simulink model "fblin_singletrack_lopez2"  (R2018b)
settings: Solver=VariableStepAuto  StartTime=0.0  StopTime=5.0  RelTol=1e-3
values from neighbouring files (symbols this model uses):
  actuation_delay = 0.09    [init_singletrack.m]
  beta_velocity_threshold = 0.05    [init_singletrack.m]
  car_param = [a, b, Cf, Cr, Iz, m]    [init_singletrack.m]
  car_state0 = [psi0, r0, beta0, x0, y0]    [init_singletrack.m]
  fblin_Ts = 0.01    [init_singletrack.m]
  meas_Ts = 0.001    [init_singletrack.m]
  P = 0.5    [init_singletrack.m]    (also in init_unicycle.m)
  psi_fir = [0.0144, 0.0439, 0.1202, 0.2025, 0.2380, 0.2025, 0.1202, 0.0439, 0.0144]    [init_singletrack.m]
  psi_noiseVar = 9e-7    (= 9e-07)    [init_singletrack.m]
  r_noiseVar = 9e-7    (= 9e-07)    [init_singletrack.m]
  vel_fir = [0.0144, 0.0295, 0.0763, 0.0823, 0.0355, -0.0355, -0.0823, -0.0763, -0.0295, -0.0144]    [init_singletrack.m]
  xy_noiseVar = 1e-8    (= 1e-08)    [init_singletrack.m]
undefined symbols (not defined in the file or in its folder): DiscIntNeverNeededParam, fblin_control_singletrack_lopez2, fblin_output_singletrack_lopez2, sigmf, singleTrack_model
libraries: simulink x1
settings Model: Creator=bascetta  LastModifiedBy=bascetta
settings DebuggingCC: LibraryContextMissingDiagnostic=none
settings SFSimCC: SimUseLocalCustomCode=off
settings RTWCC: RTWUseLocalCustomCode=off

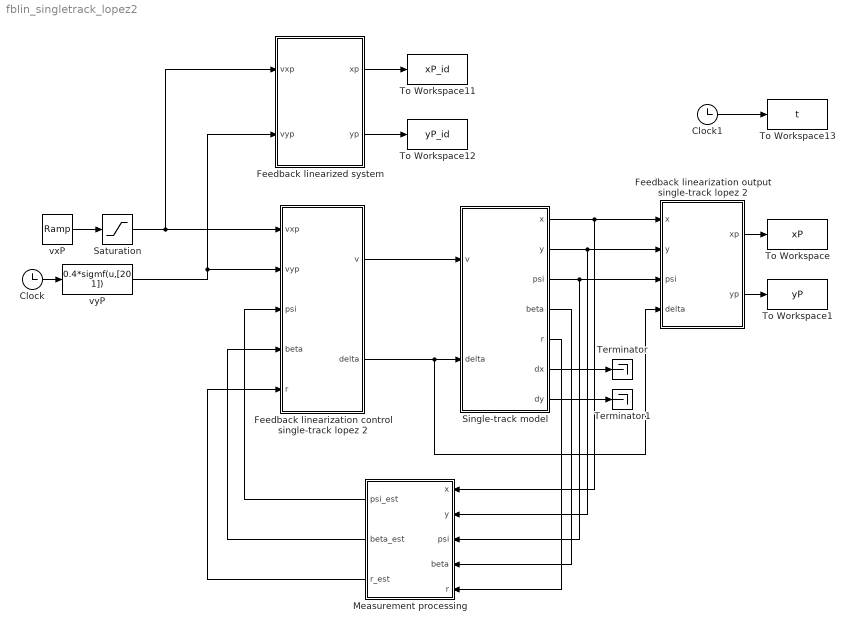
== system fblin_singletrack_lopez2 ==
  Clock : Clock
  Clock1 : Clock
  Feedback linearization control single-track lopez 2 : Subsystem  mask{car_parameters=car_param, P_dist=P, Ts=fblin_Ts}
      mask prompts: car_parameters "Car parameters"; P_dist "Distance of point P"; Ts "Sampling time"
  Feedback linearization output single-track lopez 2 : Subsystem  mask{car_parameters=car_param, P_dist=P}
      mask prompts: car_parameters "Car parameters"; P_dist "Distance of point P"
  Feedback linearized system : Subsystem  mask{car_parameters=car_param, car_initial_state=car_state0, P_dist=P}
      mask prompts: car_parameters "Car parameters"; car_initial_state "Car initial state"; P_dist "Distance of point P"
  Measurement processing : Subsystem
  Saturation : Saturate  UpperLimit=0.4  LowerLimit=0.0
  Single-track model : Subsystem  mask{car_parameters=car_param, actuation_delay=actuation_delay}
      mask prompts: car_parameters "Car parameters"; actuation_delay "Actuation delay"
  Terminator : Terminator
  Terminator1 : Terminator
  To Workspace : ToWorkspace  VariableName=xP  SampleTime=meas_Ts
      settings: Save2DSignal=2-D array (concatenate along first dimension)
  To Workspace1 : ToWorkspace  VariableName=yP  SampleTime=meas_Ts
      settings: Save2DSignal=2-D array (concatenate along first dimension)
  To Workspace11 : ToWorkspace  VariableName=xP_id  SampleTime=meas_Ts
      settings: Save2DSignal=2-D array (concatenate along first dimension)
  To Workspace12 : ToWorkspace  VariableName=yP_id  SampleTime=meas_Ts
      settings: Save2DSignal=2-D array (concatenate along first dimension)
  To Workspace13 : ToWorkspace  VariableName=t  SampleTime=meas_Ts
      settings: Save2DSignal=2-D array (concatenate along first dimension)
  vxP : simulink/Sources/Ramp  slope=0.8  start=0  InitialOutput=0
  vyP : MATLABFcn  MATLABFcn=0.4*sigmf(u,[20 1])
  wires:
  Saturation/1 -> Feedback linearization control single-track lopez 2/1(vxp), Feedback linearized system/1(vxp)
  Feedback linearization output single-track lopez 2/2(yp) -> To Workspace1/1
  Feedback linearization output single-track lopez 2/1(xp) -> To Workspace/1
  Feedback linearized system/1(xp) -> To Workspace11/1
  Feedback linearized system/2(yp) -> To Workspace12/1
  Clock1/1 -> To Workspace13/1
  Single-track model/1(x) -> Measurement processing/1(x), Feedback linearization output single-track lopez 2/1(x)
  Single-track model/2(y) -> Measurement processing/2(y), Feedback linearization output single-track lopez 2/2(y)
  Single-track model/3(psi) -> Measurement processing/3(psi), Feedback linearization output single-track lopez 2/3(psi)
  Single-track model/4(beta) -> Measurement processing/4(beta)
  Feedback linearization control single-track lopez 2/2(delta) -> Feedback linearization output single-track lopez 2/4(delta), Single-track model/2(delta)
  Feedback linearization control single-track lopez 2/1(v) -> Single-track model/1(v)
  Single-track model/5(r) -> Measurement processing/5(r)
  Measurement processing/1(psi_est) -> Feedback linearization control single-track lopez 2/3(psi)
  Measurement processing/2(beta_est) -> Feedback linearization control single-track lopez 2/4(beta)
  Measurement processing/3(r_est) -> Feedback linearization control single-track lopez 2/5(r)
  Single-track model/7(dy) -> Terminator1/1
  Single-track model/6(dx) -> Terminator/1
  vxP/1 -> Saturation/1
  Clock/1 -> vyP/1
  vyP/1 -> Feedback linearized system/2(vyp), Feedback linearization control single-track lopez 2/2(vyp)

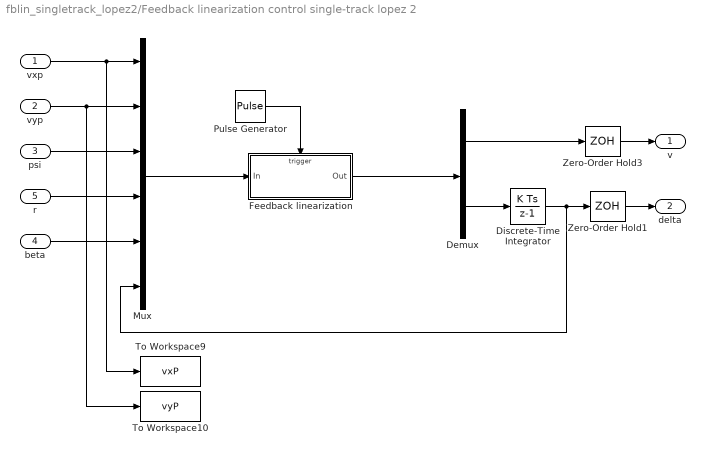
== system fblin_singletrack_lopez2/Feedback linearization control single-track lopez 2 ==
  vxp : Inport
  vyp : Inport  Port=2
  psi : Inport  Port=3
  beta : Inport  Port=4
  r : Inport  Port=5
  Demux : Demux  Outputs=2
  Discrete-Time Integrator : DiscreteIntegrator  SampleTime=Ts  ICPrevOutput=DiscIntNeverNeededParam  ICPrevScaledInput=DiscIntNeverNeededParam
  Feedback linearization : Subsystem  TreatAsAtomicUnit=on
  Mux : Mux  Inputs=6
  Pulse Generator : DiscretePulseGenerator  PulseType=Time based  Period=Ts  PulseWidth=50
  To Workspace10 : ToWorkspace  VariableName=vyP  SampleTime=meas_Ts
      settings: Save2DSignal=2-D array (concatenate along first dimension)
  To Workspace9 : ToWorkspace  VariableName=vxP  SampleTime=meas_Ts
      settings: Save2DSignal=2-D array (concatenate along first dimension)
  Zero-Order Hold1 : ZeroOrderHold  SampleTime=Ts
  Zero-Order Hold3 : ZeroOrderHold  SampleTime=Ts
  v : Outport
  delta : Outport  Port=2
  wires:
  vyp/1 -> To Workspace10/1, Mux/2
  Demux/1 -> Zero-Order Hold3/1
  vxp/1 -> To Workspace9/1, Mux/1
  psi/1 -> Mux/3
  beta/1 -> Mux/5
  r/1 -> Mux/4
  Zero-Order Hold3/1 -> v/1
  Discrete-Time Integrator/1 -> Mux/6, Zero-Order Hold1/1
  Zero-Order Hold1/1 -> delta/1
  Feedback linearization/1(Out) -> Demux/1
  Mux/1 -> Feedback linearization/1(In)
  Pulse Generator/1 -> Feedback linearization/Trigger
  Demux/2 -> Discrete-Time Integrator/1

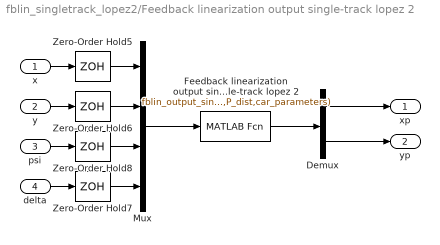
== system fblin_singletrack_lopez2/Feedback linearization output single-track lopez 2 ==
  x : Inport
  y : Inport  Port=2
  psi : Inport  Port=3
  delta : Inport  Port=4
  Demux : Demux  Outputs=2
  Feedback linearization output single-track lopez 2 : MATLABFcn  MATLABFcn=fblin_output_singletrack_lopez2(u(1),u(2),u(3),u(4),P_dist,car_parameters)  OutputDimensions=2
  Mux : Mux
  Zero-Order Hold{5..8} (4 alike) : ZeroOrderHold  SampleTime=fblin_Ts
  xp : Outport
  yp : Outport  Port=2
  wires:
  y/1 -> Zero-Order Hold6/1
  Demux/2 -> yp/1
  Feedback linearization output single-track lopez 2/1 -> Demux/1
  Demux/1 -> xp/1
  Mux/1 -> Feedback linearization output single-track lopez 2/1
  x/1 -> Zero-Order Hold5/1
  delta/1 -> Zero-Order Hold7/1
  psi/1 -> Zero-Order Hold8/1
  Zero-Order Hold5/1 -> Mux/1
  Zero-Order Hold6/1 -> Mux/2
  Zero-Order Hold7/1 -> Mux/4
  Zero-Order Hold8/1 -> Mux/3

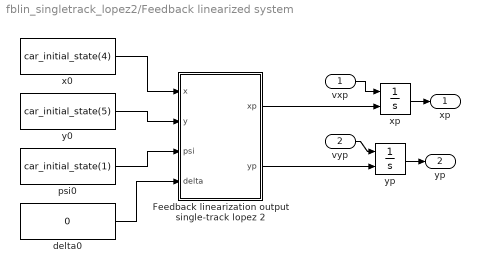
== system fblin_singletrack_lopez2/Feedback linearized system ==
  vxp : Inport
  vyp : Inport  Port=2
  " xp " : Integrator  InitialConditionSource=external  InitialCondition=car_state0(4)
  " yp " : Integrator  InitialConditionSource=external  InitialCondition=car_state0(5)
  Feedback linearization output single-track lopez 2 : Subsystem  mask{car_parameters=car_parameters, P_dist=P_dist}
      mask prompts: car_parameters "Car parameters"; P_dist "Distance of point P"
  delta0 : Constant  Value=0
  psi0 : Constant  Value=car_initial_state(1)
  x0 : Constant  Value=car_initial_state(4)
  y0 : Constant  Value=car_initial_state(5)
  xp : Outport
  yp : Outport  Port=2
  wires:
  vyp/1 -> " yp "/1
  vxp/1 -> " xp "/1
  " yp "/1 -> yp/1
  " xp "/1 -> xp/1
  x0/1 -> Feedback linearization output single-track lopez 2/1(x)
  y0/1 -> Feedback linearization output single-track lopez 2/2(y)
  psi0/1 -> Feedback linearization output single-track lopez 2/3(psi)
  delta0/1 -> Feedback linearization output single-track lopez 2/4(delta)
  Feedback linearization output single-track lopez 2/1(xp) -> " xp "/2
  Feedback linearization output single-track lopez 2/2(yp) -> " yp "/2

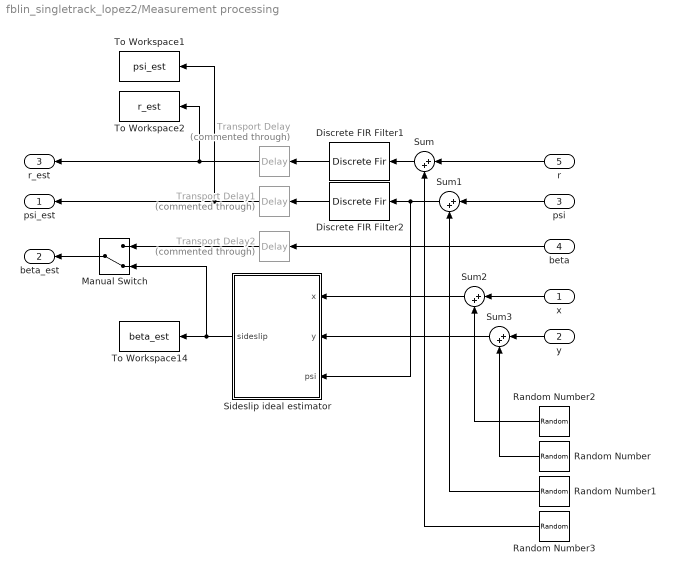
== system fblin_singletrack_lopez2/Measurement processing ==
  x : Inport
  y : Inport  Port=2
  psi : Inport  Port=3
  beta : Inport  Port=4
  r : Inport  Port=5
  Discrete FIR Filter1 : DiscreteFir  Coefficients=psi_fir  SampleTime=fblin_Ts
  Discrete FIR Filter2 : DiscreteFir  Coefficients=psi_fir  SampleTime=fblin_Ts
  Manual Switch : ManualSwitch  CurrentSetting=0
  Random Number : RandomNumber  Variance=xy_noiseVar  Seed=1
  Random Number1 : RandomNumber  Variance=psi_noiseVar  Seed=2
  Random Number2 : RandomNumber  Variance=xy_noiseVar
  Random Number3 : RandomNumber  Variance=r_noiseVar  Seed=2
  Sideslip ideal estimator : Subsystem
  Sum{,1..3} (4 alike) : Sum  Inputs=|++
  To Workspace1 : ToWorkspace  VariableName=psi_est  SampleTime=meas_Ts
      settings: Save2DSignal=2-D array (concatenate along first dimension)
  To Workspace14 : ToWorkspace  VariableName=beta_est  SampleTime=meas_Ts
      settings: Save2DSignal=2-D array (concatenate along first dimension)
  To Workspace2 : ToWorkspace  VariableName=r_est  SampleTime=meas_Ts
      settings: Save2DSignal=2-D array (concatenate along first dimension)
  Transport Delay : TransportDelay  Commented=through  DelayTime=0.02
  Transport Delay1 : TransportDelay  Commented=through  DelayTime=0.02
  Transport Delay2 : TransportDelay  Commented=through  DelayTime=0.02
  psi_est : Outport
  beta_est : Outport  Port=2
  r_est : Outport  Port=3
  wires:
  beta/1 -> Transport Delay2/1
  Transport Delay2/1 -> Manual Switch/1
  Discrete FIR Filter1/1 -> Transport Delay/1
  Discrete FIR Filter2/1 -> Transport Delay1/1
  Manual Switch/1 -> beta_est/1
  Sideslip ideal estimator/1(sideslip) -> Manual Switch/2, To Workspace14/1
  Transport Delay/1 -> To Workspace2/1, r_est/1
  Transport Delay1/1 -> To Workspace1/1, psi_est/1
  Random Number1/1 -> Sum1/2
  Random Number3/1 -> Sum/2
  Random Number2/1 -> Sum2/2
  Random Number/1 -> Sum3/2
  x/1 -> Sum2/1
  Sum2/1 -> Sideslip ideal estimator/1(x)
  psi/1 -> Sum1/1
  Sum1/1 -> Sideslip ideal estimator/3(psi), Discrete FIR Filter2/1
  Sum/1 -> Discrete FIR Filter1/1
  r/1 -> Sum/1
  y/1 -> Sum3/1
  Sum3/1 -> Sideslip ideal estimator/2(y)

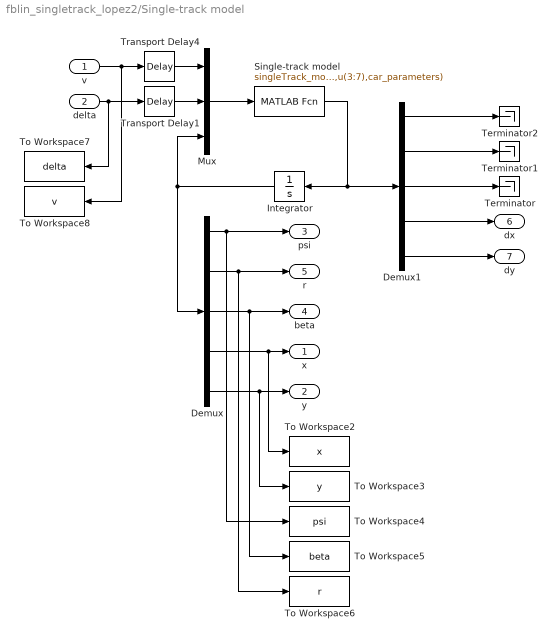
== system fblin_singletrack_lopez2/Single-track model ==
  v : Inport
  delta : Inport  Port=2
  Demux : Demux  Outputs=5
  Demux1 : Demux  Outputs=5
  Integrator : Integrator  InitialCondition=car_state0
  Mux : Mux  Inputs=3
  Single-track model : MATLABFcn  MATLABFcn=singleTrack_model(u(1:2),u(3:7),car_parameters)  OutputDimensions=5
  Terminator : Terminator
  Terminator1 : Terminator
  Terminator2 : Terminator
  To Workspace2 : ToWorkspace  VariableName=x  SampleTime=meas_Ts
      settings: Save2DSignal=2-D array (concatenate along first dimension)
  To Workspace3 : ToWorkspace  VariableName=y  SampleTime=meas_Ts
      settings: Save2DSignal=2-D array (concatenate along first dimension)
  To Workspace4 : ToWorkspace  VariableName=psi  SampleTime=meas_Ts
      settings: Save2DSignal=2-D array (concatenate along first dimension)
  To Workspace5 : ToWorkspace  VariableName=beta  SampleTime=meas_Ts
      settings: Save2DSignal=2-D array (concatenate along first dimension)
  To Workspace6 : ToWorkspace  VariableName=r  SampleTime=meas_Ts
      settings: Save2DSignal=2-D array (concatenate along first dimension)
  To Workspace7 : ToWorkspace  VariableName=delta  SampleTime=meas_Ts
      settings: Save2DSignal=2-D array (concatenate along first dimension)
  To Workspace8 : ToWorkspace  VariableName=v  SampleTime=meas_Ts
      settings: Save2DSignal=2-D array (concatenate along first dimension)
  Transport Delay1 : TransportDelay  DelayTime=actuation_delay
  Transport Delay4 : TransportDelay  DelayTime=actuation_delay
  x : Outport
  y : Outport  Port=2
  psi : Outport  Port=3
  beta : Outport  Port=4
  r : Outport  Port=5
  dx : Outport  Port=6
  dy : Outport  Port=7
  wires:
  Integrator/1 -> Demux/1, Mux/3
  Single-track model/1 -> Demux1/1, Integrator/1
  delta/1 -> To Workspace7/1, Transport Delay1/1
  Demux/4 -> To Workspace2/1, x/1
  Mux/1 -> Single-track model/1
  Demux/5 -> To Workspace3/1, y/1
  Demux/3 -> To Workspace5/1, beta/1
  v/1 -> To Workspace8/1, Transport Delay4/1
  Demux/2 -> To Workspace6/1, r/1
  Demux/1 -> To Workspace4/1, psi/1
  Demux1/5 -> dy/1
  Demux1/4 -> dx/1
  Demux1/2 -> Terminator1/1
  Demux1/3 -> Terminator/1
  Demux1/1 -> Terminator2/1
  Transport Delay4/1 -> Mux/1
  Transport Delay1/1 -> Mux/2

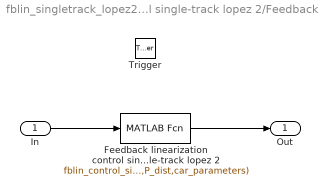
== system fblin_singletrack_lopez2/Feedback linearization control single-track lopez 2/Feedback linearization ==
  In : Inport
  Trigger : TriggerPort  VariantControl=Variant
  Feedback linearization control single-track lopez 2 : MATLABFcn  MATLABFcn=fblin_control_singletrack_lopez2(u(1),u(2),u(3),u(4),u(5),u(6),P_dist,car_parameters)  OutputDimensions=2
  Out : Outport
  wires:
  In/1 -> Feedback linearization control single-track lopez 2/1
  Feedback linearization control single-track lopez 2/1 -> Out/1

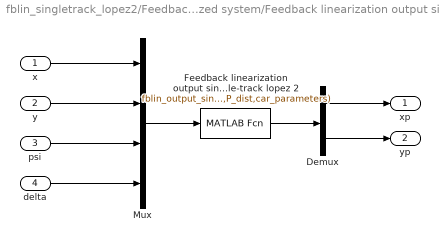
== system fblin_singletrack_lopez2/Feedback linearized system/Feedback linearization output single-track lopez 2 ==
  x : Inport
  y : Inport  Port=2
  psi : Inport  Port=3
  delta : Inport  Port=4
  Demux : Demux  Outputs=2
  Feedback linearization output single-track lopez 2 : MATLABFcn  MATLABFcn=fblin_output_singletrack_lopez2(u(1),u(2),u(3),u(4),P_dist,car_parameters)  OutputDimensions=2
  Mux : Mux
  xp : Outport
  yp : Outport  Port=2
  wires:
  Demux/2 -> yp/1
  Feedback linearization output single-track lopez 2/1 -> Demux/1
  Demux/1 -> xp/1
  Mux/1 -> Feedback linearization output single-track lopez 2/1
  x/1 -> Mux/1
  y/1 -> Mux/2
  delta/1 -> Mux/4
  psi/1 -> Mux/3

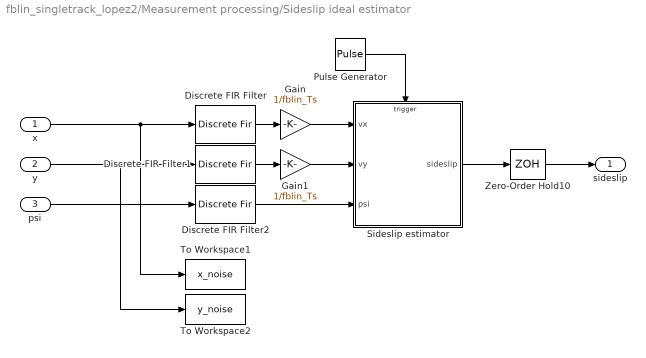
== system fblin_singletrack_lopez2/Measurement processing/Sideslip ideal estimator ==
  x : Inport
  y : Inport  Port=2
  psi : Inport  Port=3
  Discrete FIR Filter : DiscreteFir  Coefficients=vel_fir  SampleTime=fblin_Ts
  Discrete FIR Filter1 : DiscreteFir  Coefficients=vel_fir  SampleTime=fblin_Ts
  Discrete FIR Filter2 : DiscreteFir  Coefficients=psi_fir  SampleTime=fblin_Ts
  Gain : Gain  Gain=1/fblin_Ts
  Gain1 : Gain  Gain=1/fblin_Ts
  Pulse Generator : DiscretePulseGenerator  PulseType=Time based  Period=fblin_Ts  PulseWidth=50
  Sideslip estimator : Subsystem  TreatAsAtomicUnit=on
  To Workspace1 : ToWorkspace  VariableName=x_noise  SampleTime=meas_Ts
      settings: Save2DSignal=2-D array (concatenate along first dimension)
  To Workspace2 : ToWorkspace  VariableName=y_noise  SampleTime=meas_Ts
      settings: Save2DSignal=2-D array (concatenate along first dimension)
  Zero-Order Hold10 : ZeroOrderHold  SampleTime=fblin_Ts
  sideslip : Outport
  wires:
  Sideslip estimator/1(sideslip) -> Zero-Order Hold10/1
  Zero-Order Hold10/1 -> sideslip/1
  Pulse Generator/1 -> Sideslip estimator/Trigger
  Discrete FIR Filter2/1 -> Sideslip estimator/3(psi)
  y/1 -> Discrete FIR Filter1/1, To Workspace2/1
  Gain/1 -> Sideslip estimator/1(vx)
  x/1 -> Discrete FIR Filter/1, To Workspace1/1
  Discrete FIR Filter/1 -> Gain/1
  Discrete FIR Filter1/1 -> Gain1/1
  Gain1/1 -> Sideslip estimator/2(vy)
  psi/1 -> Discrete FIR Filter2/1

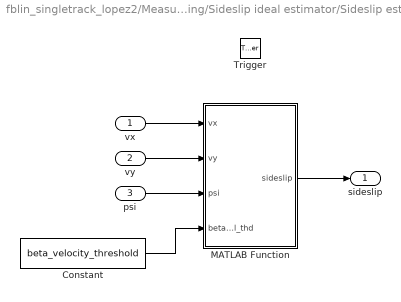
== system fblin_singletrack_lopez2/Measurement processing/Sideslip ideal estimator/Sideslip estimator ==
  vx : Inport
  vy : Inport  Port=2
  psi : Inport  Port=3
  Trigger : TriggerPort  VariantControl=Variant
  Constant : Constant  Value=beta_velocity_threshold
  MATLAB Function : MATLAB Function  TreatAsAtomicUnit=on
  sideslip : Outport
  wires:
  MATLAB Function/1(sideslip) -> sideslip/1
  vx/1 -> MATLAB Function/1(vx)
  psi/1 -> MATLAB Function/3(psi)
  vy/1 -> MATLAB Function/2(vy)
  Constant/1 -> MATLAB Function/4(beta_vel_thd)

== matlab function fblin_singletrack_lopez2/Measurement processing/Sideslip ideal estimator/Sideslip estimator/MATLAB Function ==
  data: vx input; sideslip output; vy input; psi input; beta_vel_thd input
function sideslip = fcn(vx,vy,psi,beta_vel_thd)

if (norm([vx,vy])<=beta_vel_thd)
    sideslip = 0;
else
    sideslip = atan2( -vx*sin(psi)+vy*cos(psi), vx*cos(psi)+vy*sin(psi) );
end
